simulink model "balancing_controller"  (R2022a)
settings: Solver=FixedStepDiscrete  StartTime=0.0  StopTime=StopTime  FixedStep=TimeStep  MaxStep=0.5  RelTol=1e-3  AbsTol=1e-3
settings Model: DataDictionary=passive_balancing_data.sldd  Creator=tshintai  LastModifiedBy=tshintai
settings SolverCC: AutoScaleAbsTol=off
settings DataIOCC: SaveOutput=off  SaveTime=off
settings OptimizationCC: DefaultParameterBehavior=Inlined  EnhancedBackFolding=on  PassReuseOutputArgsAs=Individual arguments  ZeroExternalMemoryAtStartup=off  ZeroInternalMemoryAtStartup=off  OptimizeBlockOrder=speed  DifferentSizesBufferReuse=on  OptimizationCustomize=off  EfficientTunableParamExpr=on
settings DebuggingCC: ParameterTunabilityLossMsg=error  UnconnectedInputMsg=warning  UnconnectedOutputMsg=warning  UnconnectedLineMsg=warning
settings SFSimCC: MATLABDynamicMemAlloc=off
settings RTWCC: SystemTargetFile=ert.tlc  TemplateMakefile=ert_default_tmf  GenerateReport=on  LaunchReport=on  GenerateCodeMetricsReport=on  DLArmComputeVersion=19.05
settings CodeAppCC: ForceParamTrailComments=on  IgnoreCustomStorageClasses=off  OperatorAnnotations=on  SimulinkDataObjDesc=on  SFDataObjDesc=on  InsertBlockDesc=on
settings ERTTargetCC: TargetLangStandard=C99 (ISO)  GenerateSampleERTMain=on  InlinedParameterPlacement=NonHierarchical  ERTCustomFileTemplate=example_file_process.tlc

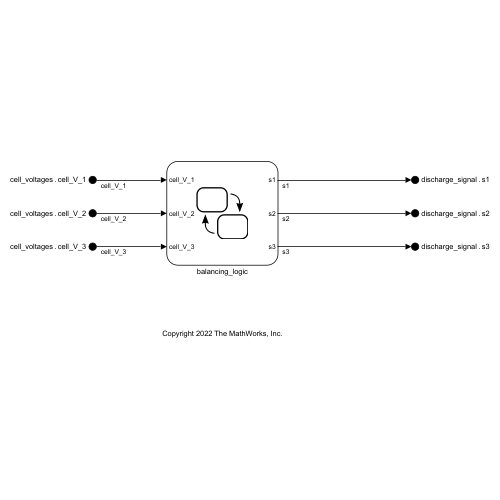
[thumbnail: Simulink's stored preview of the top-level diagram]
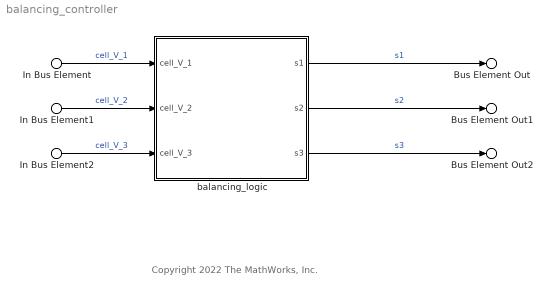
== system balancing_controller ==
  note: Copyright 2022 The MathWorks, Inc.
  In Bus Element : Inport  PortName=cell_voltages  Element=cell_V_1
  In Bus Element1 : Inport  PortName=cell_voltages  Element=cell_V_2
  In Bus Element2 : Inport  PortName=cell_voltages  Element=cell_V_3
  balancing_logic : Stateflow chart  TreatAsAtomicUnit=on  VariantControl=(default)
  Bus Element Out : Outport  PortName=discharge_signal  Element=s1
  Bus Element Out1 : Outport  PortName=discharge_signal  Element=s2
  Bus Element Out2 : Outport  PortName=discharge_signal  Element=s3
  wires:
  balancing_logic/2(s2) -> Bus Element Out1/1  "s2"
  balancing_logic/3(s3) -> Bus Element Out2/1  "s3"
  balancing_logic/1(s1) -> Bus Element Out/1  "s1"
  In Bus Element/1 -> balancing_logic/1(cell_V_1)  "cell_V_1"
  In Bus Element1/1 -> balancing_logic/2(cell_V_2)  "cell_V_2"
  In Bus Element2/1 -> balancing_logic/3(cell_V_3)  "cell_V_3"

== stateflow chart balancing_controller/balancing_logic ==
  settings: updateMethod=DISCRETE
  state init
    entry:
    s1 = DISCHARGE_FLAG.OFF;
    s2 = DISCHARGE_FLAG.OFF;
    s3 = DISCHARGE_FLAG.OFF;
  state finish
    entry:
    s1 = DISCHARGE_FLAG.OFF;
    s2 = DISCHARGE_FLAG.OFF;
    s3 = DISCHARGE_FLAG.OFF;
  state balancing
    du: sort_V = ord(cell_V_1, cell_V_2, cell_V_3);
    state s1_s2
      en:
      s1 = DISCHARGE_FLAG.ON;
      s2 = DISCHARGE_FLAG.ON;
      s3 = DISCHARGE_FLAG.OFF;
      ex:
      s1 = DISCHARGE_FLAG.OFF;
      s2 = DISCHARGE_FLAG.OFF;
      s3 = DISCHARGE_FLAG.OFF;
    state s1_s3
      en:
      s1 = DISCHARGE_FLAG.ON;
      s2 = DISCHARGE_FLAG.OFF;
      s3 = DISCHARGE_FLAG.ON;
      ex:
      s1 = DISCHARGE_FLAG.OFF;
      s2 = DISCHARGE_FLAG.OFF;
      s3 = DISCHARGE_FLAG.OFF;
    state s2_s3
      en:
      s1 = DISCHARGE_FLAG.OFF;
      s2 = DISCHARGE_FLAG.ON;
      s3 = DISCHARGE_FLAG.ON;
      ex:
      s1 = DISCHARGE_FLAG.OFF;
      s2 = DISCHARGE_FLAG.OFF;
      s3 = DISCHARGE_FLAG.OFF;
    (default) -> (junction 382) : {
        | sort_V = ord(cell_V_1, cell_V_2, cell_V_3);
        | }
    (junction 382) -> (junction 422) [order 1] : % cell#1 lowest
        | [
        | sort_V(1) == 1
        | ]
    (junction 382) -> (junction 428) [order 2]
    (junction 422) -> s2_s3
    (junction 428) -> (junction 429) [order 1] : % cell#2 lowest
        | [
        | sort_V(1) == 2
        | ]
    (junction 428) -> s1_s2 [order 2] : % cell#3 lowest
    (junction 429) -> s1_s3
    s1_s2 -> s1_s3 [order 1] : [
        | sort_V(1) == 2
        | ]
    s1_s3 -> s2_s3 [order 2] : [
        | sort_V(1) == 1
        | ]
    s1_s3 -> s1_s2 [order 1] : [
        | sort_V(1) == 3
        | ]
    s2_s3 -> s1_s3 [order 1] : [
        | sort_V(1) == 2
        | ]
    s1_s2 -> (junction 414) [order 2] : [
        | sort_V(1) == 1
        | ]
    (junction 415) -> s1_s2
    s2_s3 -> (junction 416) [order 2] : [
        | sort_V(1) == 3
        | ]
    (junction 417) -> s2_s3
    (junction 416) -> (junction 415)
    (junction 414) -> (junction 417)
  (default) -> init
  init -> balancing : [
      | abs(max([cell_V_1, cell_V_2, cell_V_3]) - ...
      |       min([cell_V_1, cell_V_2, cell_V_3])) ...
      | > delta_V
      | ]
  finish -> balancing : [
      | abs(max([cell_V_1, cell_V_2, cell_V_3]) - ...
      |       min([cell_V_1, cell_V_2, cell_V_3])) ...
      | > delta_V ...
      | && ...
      | after(1,sec)
      | ]
  balancing -> finish : [
      | abs(max([cell_V_1, cell_V_2, cell_V_3]) - ...
      |       min([cell_V_1, cell_V_2, cell_V_3])) ...
      | < delta_V
      | ]
  data: a function_input; b function_input; c function_input; p function_output; cell_V_1 input; cell_V_2 input; cell_V_3 input; s1 output Enum: DISCHARGE_FLAG; s2 output Enum: DISCHARGE_FLAG; s3 output Enum: DISCHARGE_FLAG; delta_V parameter; sort_V local =[1,2,3]
  function p = ord(a,b,c):
    | function p = ord(a,b,c)
    | [~,p] = sort([a,b,c],'ascend');
